simulink model "SupportedDeltaModelElements"  (Simulink 7.8)
settings: Solver=ode45  StartTime=0.0  StopTime=10.0  RelTol=1e-3
settings Model: Creator=Arne Haber  LastModifiedBy=Arne Haber

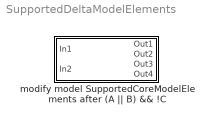
== system SupportedDeltaModelElements ==
  modify model SupportedCoreModelElements after (A || B) && !C : Subsystem

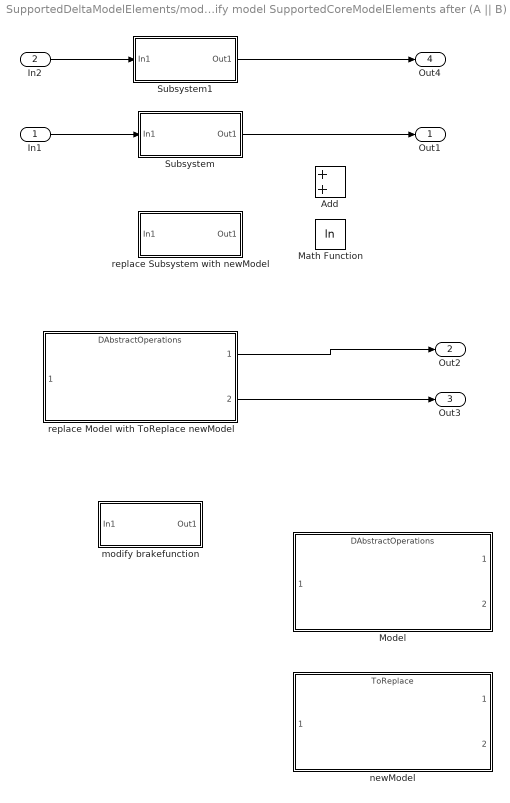
== system SupportedDeltaModelElements/modify model SupportedCoreModelElements after (A || B) && !C ==
  In1 : Inport
  In2 : Inport  Port=2
  Add : Sum
  Math Function : Math  Operator=log  SaturateOnIntegerOverflow=on
  Model : ModelReference  ModelNameDialog=DAbstractOperations  SimulationMode=Normal  ModelReferenceVersion=1.8  CopyOfModelName=DAbstractOperations  DefaultDataLogging=on
  Subsystem : Subsystem
  Subsystem1 : Subsystem
  modify brakefunction : Subsystem
  newModel : ModelReference  ModelNameDialog=ToReplace  SimulationMode=Normal  ModelReferenceVersion=1.1  CopyOfModelName=ToReplace  DefaultDataLogging=on
  replace Model with ToReplace newModel : ModelReference  ModelNameDialog=DAbstractOperations  SimulationMode=Normal  ModelReferenceVersion=1.8  CopyOfModelName=DAbstractOperations  DefaultDataLogging=on
  replace Subsystem with newModel : Subsystem
  Out1 : Outport
  Out2 : Outport  Port=2
  Out3 : Outport  Port=3
  Out4 : Outport  Port=4
  wires:
  In1/1 -> Subsystem/1(In1)
  Subsystem/1(Out1) -> Out1/1
  In2/1 -> Subsystem1/1(In1)
  Subsystem1/1(Out1) -> Out4/1
  replace Model with ToReplace newModel/1 -> Out2/1
  replace Model with ToReplace newModel/2 -> Out3/1

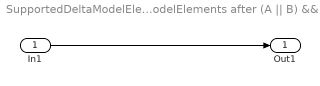
== system SupportedDeltaModelElements/modify model SupportedCoreModelElements after (A || B) && !C/Subsystem ==
  In1 : Inport
  Out1 : Outport
  wires:
  In1/1 -> Out1/1

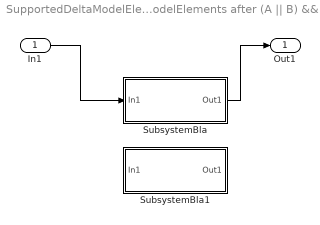
== system SupportedDeltaModelElements/modify model SupportedCoreModelElements after (A || B) && !C/Subsystem1 ==
  In1 : Inport
  SubsystemBla : Subsystem
  SubsystemBla1 : Subsystem
  Out1 : Outport
  wires:
  In1/1 -> SubsystemBla/1(In1)
  SubsystemBla/1(Out1) -> Out1/1

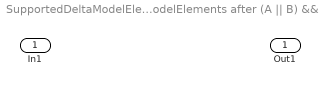
== system SupportedDeltaModelElements/modify model SupportedCoreModelElements after (A || B) && !C/modify brakefunction ==
  In1 : Inport
  Out1 : Outport

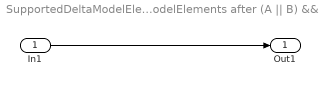
== system SupportedDeltaModelElements/modify model SupportedCoreModelElements after (A || B) && !C/replace Subsystem with newModel ==
  In1 : Inport
  Out1 : Outport
  wires:
  In1/1 -> Out1/1

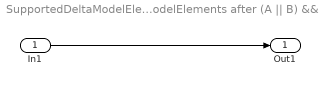
== system SupportedDeltaModelElements/modify model SupportedCoreModelElements after (A || B) && !C/Subsystem1/SubsystemBla ==
  In1 : Inport
  Out1 : Outport
  wires:
  In1/1 -> Out1/1

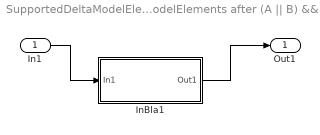
== system SupportedDeltaModelElements/modify model SupportedCoreModelElements after (A || B) && !C/Subsystem1/SubsystemBla1 ==
  In1 : Inport
  InBla1 : Subsystem
  Out1 : Outport
  wires:
  In1/1 -> InBla1/1(In1)
  InBla1/1(Out1) -> Out1/1

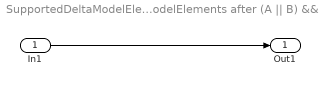
== system SupportedDeltaModelElements/modify model SupportedCoreModelElements after (A || B) && !C/Subsystem1/SubsystemBla1/InBla1 ==
  In1 : Inport
  Out1 : Outport
  wires:
  In1/1 -> Out1/1
